simulink model "DriveCycle"  (R2019b)
settings: Solver=FixedStepAuto  StartTime=0  StopTime=10  FixedStep=0.1  RelTol=1e-3  EnableMultiTasking=on
libraries: simulink x2, arduinolib x2, autolibshared x1
settings Model: SILPILModeSetting=veronly  ExtModeTrigDuration=2  Creator=snehi  LastModifiedBy=snehi
settings OptimizationCC: EnhancedBackFolding=on  PassReuseOutputArgsAs=Individual arguments  ZeroExternalMemoryAtStartup=off  ZeroInternalMemoryAtStartup=off  MaxStackSize=64  OptimizeBlockOrder=speed  DifferentSizesBufferReuse=on  OptimizationCustomize=off  EfficientTunableParamExpr=on
settings DebuggingCC: ParameterPrecisionLossMsg=none  ParameterTunabilityLossMsg=error
settings HardwareCC: ProdBitPerInt=16  ProdBitPerPointer=16  ProdBitPerSizeT=16  ProdBitPerPtrDiffT=16  ProdLargestAtomicFloat=None  ProdWordSize=8  ProdHWDeviceType=Atmel->AVR  UseEmbeddedCoderFeatures=off  UseSimulinkCoderFeatures=off
settings SFSimCC: MATLABDynamicMemAlloc=off
settings RTWCC: SystemTargetFile=ert.tlc  HardwareBoard=Arduino Uno  TLCOptions=-aInlineSetEventsForThisBaseRateFcn=TLC_FALSE -aSuppressMultiTaskScheduler=TLC_FALSE -aRateBasedStepFcn=1  TemplateMakefile=ert_default_tmf  GenerateReport=on  Toolchain=Arduino AVR  BuildConfiguration=Faster Runs  IncludeHyperlinkInReport=on  LaunchReport=on  GenerateTraceInfo=on  GenerateTraceReport=on  GenerateTraceReportSl=on  GenerateTraceReportSf=on  GenerateTraceReportEml=on
settings CodeAppCC: ForceParamTrailComments=on  IgnoreCustomStorageClasses=off  OperatorAnnotations=on  SimulinkDataObjDesc=on  SFDataObjDesc=on  InsertBlockDesc=on
settings ERTTargetCC: SupportContinuousTime=on  SupportNonInlinedSFcns=on  SupportVariableSizeSignals=on  ExtModeStaticAllocSize=250

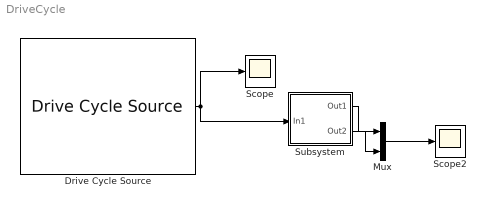
== system DriveCycle ==
  Drive Cycle Source : autolibshared/Drive Cycle Source  cycleVar=.mat, .xls, .xlsx or .txt file  fileVar=C:\Users\snehi\Desktop\Spoiler\DriveCycle.xlsx  tfinal="9  seconds"  cycleRepeat=off  outAccPort=off  outGearPort=off  gearList=No gear data  t_wot1=5  xdot_woto=1  xdot_wot1=30  t_wot2=7  xdot_wot2=50  t_wotend=8  srcUnit=m/s  outUnit=m/s  srcAccUnit=m/s/s  outAccUnit=m/s^2  dt=0.1  aMode=2
      settings: SourceProductName=Powertrain Blockset  SourceProductBaseCode=PW
  Mux : Mux  Inputs=2
  Scope : Scope
  Scope2 : Scope
  Subsystem : Subsystem
  wires:
  Subsystem/2(Out2) -> Mux/2
  Mux/1 -> Scope2/1
  Subsystem/1(Out1) -> Mux/1
  Drive Cycle Source/1 -> Scope/1, Subsystem/1(In1)

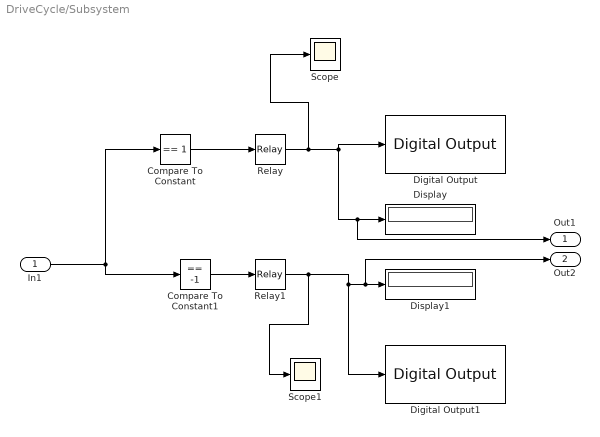
== system DriveCycle/Subsystem ==
  In1 : Inport
  Compare To Constant : simulink/Logic and Bit Operations/Compare To Constant  relop===  const=1  OutDataTypeStr=boolean
  Compare To Constant1 : simulink/Logic and Bit Operations/Compare To Constant  relop===  const=-1  OutDataTypeStr=boolean
  Digital Output : arduinolib/Digital Output  pinNumber=9  blockPlatform=arduino
  Digital Output1 : arduinolib/Digital Output  pinNumber=10  blockPlatform=arduino
  Display : Display
  Display1 : Display
  Relay : Relay
  Relay1 : Relay  OutDataTypeStr=Inherit: Inherit via back propagation
  Scope : Scope
  Scope1 : Scope
  Out1 : Outport
  Out2 : Outport  Port=2
  wires:
  Relay/1 -> Scope/1, Digital Output/1, Out1/1, Display/1
  Relay1/1 -> Scope1/1, Out2/1, Display1/1, Digital Output1/1
  Compare To Constant/1 -> Relay/1
  Compare To Constant1/1 -> Relay1/1
  In1/1 -> Compare To Constant1/1, Compare To Constant/1
